simulink model "unifiedModelEdit"  (R2023b)
settings: Solver=FixedStepAuto  StartTime=0.0  StopTime=inf  RelTol=1e-3  EnableMultiTasking=on
libraries: vexarmcortexlib x25, vexcommonlib x6
settings Model: Creator=carol  LastModifiedBy=behja
settings SolverCC: AutoInsertRateTranBlk=on
settings DataIOCC: LimitDataPoints=on  SignalLoggingSaveFormat=ModelDataLogs  ReturnWorkspaceOutputs=off
settings OptimizationCC: ExpressionDepthLimit=2147483647  LifeSpan=Inf  MaxStackSize=64  EfficientTunableParamExpr=on
settings DebuggingCC: UnderspecifiedInitializationDetection=Classic  MergeDetectMultiDrivingBlocksExec=none  InheritedTsInSrcMsg=none  FcnCallInpInsideContextMsg=warning  StateNameClashWarn=warning  SFUnexpectedBacktrackingDiag=warning  SFNoUnconditionalDefaultTransitionDiag=warning  SFExecutionAtInitializationDiag=none  ArithmeticOperatorsInVariantConditions=warning
settings HardwareCC: ProdBitPerPointer=32  ProdBitPerSizeT=32  ProdBitPerPtrDiffT=32  ProdLargestAtomicInteger=Long  ProdLargestAtomicFloat=Double  ProdIntDivRoundTo=Undefined  ProdWordSize=32  ProdHWDeviceType=ARM Compatible->ARM Cortex
settings ModelReferenceCC: EnableRefExpFcnMdlSchedulingChecks=on  PropagateSignalLabelsOutOfModel=off
settings SFSimCC: MATLABDynamicMemAlloc=off  CustomCodeUndefinedFunction=UseInterfaceOnly
settings RTWCC: Description=Embedded Coder  SystemTargetFile=ert.tlc  HardwareBoard=ARM Cortex-based VEX Microcontroller  TemplateMakefile=ert_default_tmf  Toolchain=GNU Tools for VEX ARM Cortex
settings CodeAppCC: IgnoreCustomStorageClasses=off  CustomSymbolStrType=$N$R$M  StateflowObjectComments=on  InternalIdentifier=Classic
settings ERTTargetCC: CodeReplacementLibrary=GCC ARM Cortex-M3  MultiwordLength=2048  ConvertIfToSwitch=off  SuppressUnreachableDefaultCases=off

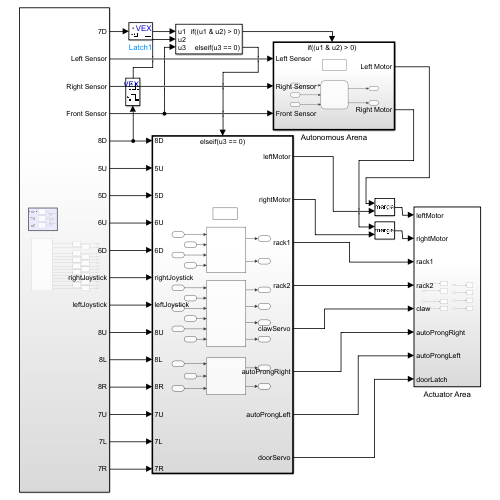
[thumbnail: Simulink's stored preview of the top-level diagram]
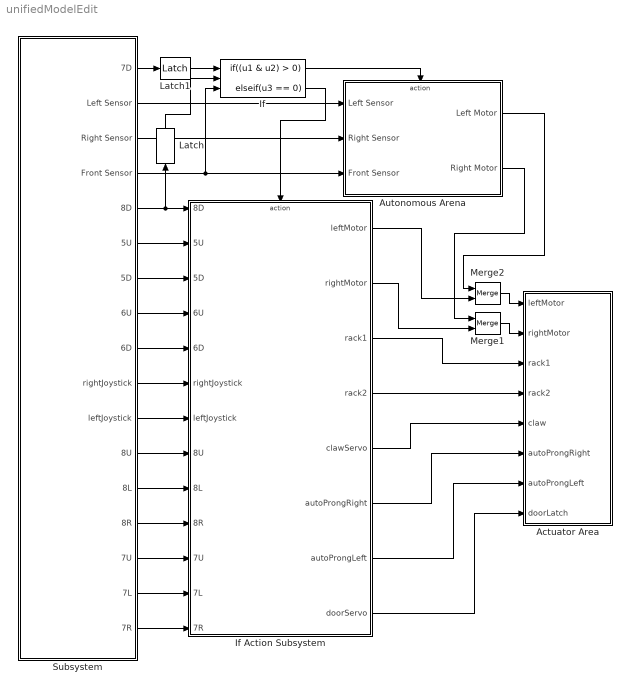
== system unifiedModelEdit ==
  Actuator Area : Subsystem
  Autonomous Arena : Subsystem  TreatAsAtomicUnit=on
  If : If  NumInputs=3  IfExpression=(u1 & u2) > 0  ElseIfExpressions=u3 == 0  ShowElse=off
  If Action Subsystem : Subsystem  TreatAsAtomicUnit=on
  Latch : vexcommonlib/Latch  output0=off  BlockPlatform=vexarmcortex
      settings: LibrarySourceBlock=vexarmcortexlib/Utilities/Latch
  Latch1 : vexcommonlib/Latch  output0=off  BlockPlatform=vexarmcortex
      settings: LibrarySourceBlock=vexarmcortexlib/Utilities/Latch
  Merge1 : Merge
  Merge2 : Merge
  Subsystem : Subsystem
  wires:
  Subsystem/3(Right Sensor) -> Autonomous Arena/2(Right Sensor)
  Subsystem/4(Front Sensor) -> If/3, Autonomous Arena/3(Front Sensor)
  If Action Subsystem/8(doorServo) -> Actuator Area/8(doorLatch)
  Subsystem/2(Left Sensor) -> Autonomous Arena/1(Left Sensor)
  Subsystem/5(8D) -> Latch/1, If Action Subsystem/1(8D)
  If Action Subsystem/5(clawServo) -> Actuator Area/5(claw)
  If Action Subsystem/3(rack1) -> Actuator Area/3(rack1)
  If Action Subsystem/6(autoProngRight) -> Actuator Area/6(autoProngRight)
  If Action Subsystem/4(rack2) -> Actuator Area/4(rack2)
  If Action Subsystem/7(autoProngLeft) -> Actuator Area/7(autoProngLeft)
  Subsystem/17(7R) -> If Action Subsystem/13(7R)
  Subsystem/16(7L) -> If Action Subsystem/12(7L)
  Subsystem/15(7U) -> If Action Subsystem/11(7U)
  Subsystem/14(8R) -> If Action Subsystem/10(8R)
  Subsystem/13(8L) -> If Action Subsystem/9(8L)
  Subsystem/12(8U) -> If Action Subsystem/8(8U)
  Subsystem/11(leftJoystick) -> If Action Subsystem/7(leftJoystick)
  Subsystem/10(rightJoystick) -> If Action Subsystem/6(rightJoystick)
  Subsystem/9(6D) -> If Action Subsystem/5(6D)
  Subsystem/8(6U) -> If Action Subsystem/4(6U)
  Subsystem/7(5D) -> If Action Subsystem/3(5D)
  Subsystem/6(5U) -> If Action Subsystem/2(5U)
  Merge1/1 -> Actuator Area/2(rightMotor)
  Merge2/1 -> Actuator Area/1(leftMotor)
  Autonomous Arena/1(Left Motor) -> Merge2/1
  If Action Subsystem/1(leftMotor) -> Merge2/2
  Autonomous Arena/2(Right Motor) -> Merge1/1
  If Action Subsystem/2(rightMotor) -> Merge1/2
  If/2 -> If Action Subsystem/Action
  If/1 -> Autonomous Arena/Action
  Latch/1 -> If/2
  Subsystem/1(7D) -> Latch1/1
  Latch1/1 -> If/1

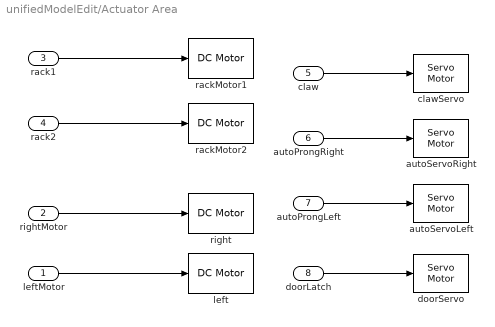
== system unifiedModelEdit/Actuator Area ==
  leftMotor : Inport
  rightMotor : Inport  Port=2
  rack1 : Inport  Port=3
  rack2 : Inport  Port=4
  claw : Inport  Port=5
  autoProngRight : Inport  Port=6
  autoProngLeft : Inport  Port=7
  doorLatch : Inport  Port=8
  autoServoLeft : vexarmcortexlib/Actuators/Servo Motor  motor=4  scaleFactor=60/127  SimulationOut=off
  autoServoRight : vexarmcortexlib/Actuators/Servo Motor  motor=7  scaleFactor=60/127  SimulationOut=off
  clawServo : vexarmcortexlib/Actuators/Servo Motor  motor=3  scaleFactor=60/127  SimulationOut=off
  doorServo : vexarmcortexlib/Actuators/Servo Motor  motor=8  scaleFactor=60/127  SimulationOut=off
  left : vexarmcortexlib/Actuators/DC Motor  motor=9  scaleFactor=1/13.5  SimulationOut=off
  rackMotor1 : vexarmcortexlib/Actuators/DC Motor  motor=5  scaleFactor=1/13.5  SimulationOut=off
  rackMotor2 : vexarmcortexlib/Actuators/DC Motor  motor=6  scaleFactor=1/13.5  SimulationOut=off
  right : vexarmcortexlib/Actuators/DC Motor  motor=2  scaleFactor=1/13.5  SimulationOut=off
  wires:
  leftMotor/1 -> left/1
  autoProngLeft/1 -> autoServoLeft/1
  rack1/1 -> rackMotor1/1
  rightMotor/1 -> right/1
  autoProngRight/1 -> autoServoRight/1
  doorLatch/1 -> doorServo/1
  claw/1 -> clawServo/1
  rack2/1 -> rackMotor2/1

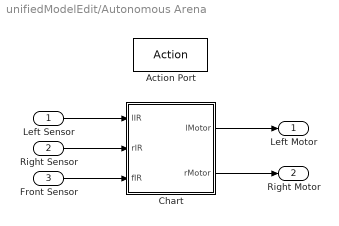
== system unifiedModelEdit/Autonomous Arena ==
  Left Sensor : Inport
  Right Sensor : Inport  Port=2
  Front Sensor : Inport  Port=3
  Action Port : ActionPort  ActionPortLabel=if((u1 & u2) > 0)
  Chart : Stateflow chart  TreatAsAtomicUnit=on
      settings: PortSchema="{\"entries\":[{\"content\":{\"sides\":[{\"content\":{\"connectorIds\":[\"In2\",\"In3\",\"In1\"]},\"type\":\"ConnectorPlacement.EquallySpacedRectSide\",\"uuid\":\"247074c7-d082-4199-9f42-5ee7f9b2f2c5\"},{\"content\":{\"connectorIds\":[\"Out1\",\"Out2\"],\"side\":\"RIGHT\"},\"type\":\"ConnectorPlacement.EquallySpacedRectSide\",\"uuid\":\"36e2493d-b1f5-4e64-901d-97da90bd168d\"},{\"content\":{\"side\":\"TOP\"},\"type\":\"ConnectorPlacement.EquallySpacedRectSide\",\"uuid\":\"46c427ed-bb7b-4aa4-a673-b474e6d6a53a\"}]},\"type\":\"ConnectorPlacement.EquallySpacedConnector\",\"uuid\":\"23614380-3184-4867-9eb4-661b2749fd08\"}],\"packageUris\":[\"http://schema.mathworks.com/mf0/Connector/R2020b\"],\"version\":\"1.0\"}"
  Left Motor : Outport
  Right Motor : Outport  Port=2
  wires:
  Left Sensor/1 -> Chart/2(lIR)
  Front Sensor/1 -> Chart/1(fIR)
  Right Sensor/1 -> Chart/3(rIR)
  Chart/1(lMotor) -> Left Motor/1
  Chart/2(rMotor) -> Right Motor/1

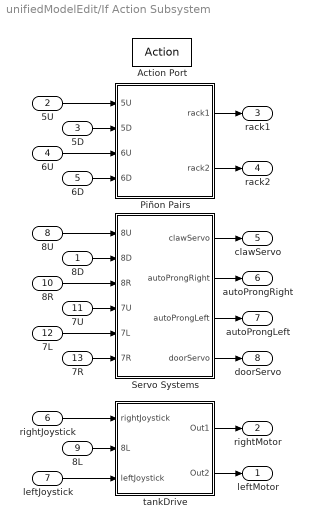
== system unifiedModelEdit/If Action Subsystem ==
  8D : Inport
  5U : Inport  Port=2
  5D : Inport  Port=3
  6U : Inport  Port=4
  6D : Inport  Port=5
  rightJoystick : Inport  Port=6
  leftJoystick : Inport  Port=7
  8U : Inport  Port=8
  8L : Inport  Port=9
  8R : Inport  Port=10
  7U : Inport  Port=11
  7L : Inport  Port=12
  7R : Inport  Port=13
  Action Port : ActionPort  ActionPortLabel=elseif(u3 == 0)
  Piñon Pairs : Subsystem
  Servo Systems : Subsystem
  tankDrive : Subsystem
  leftMotor : Outport
  rightMotor : Outport  Port=2
  rack1 : Outport  Port=3
  rack2 : Outport  Port=4
  clawServo : Outport  Port=5
  autoProngRight : Outport  Port=6
  autoProngLeft : Outport  Port=7
  doorServo : Outport  Port=8
  wires:
  Servo Systems/2(autoProngRight) -> autoProngRight/1
  Servo Systems/4(doorServo) -> doorServo/1
  Servo Systems/3(autoProngLeft) -> autoProngLeft/1
  Servo Systems/1(clawServo) -> clawServo/1
  7U/1 -> Servo Systems/4(7U)
  8D/1 -> Servo Systems/2(8D)
  Piñon Pairs/1(rack1) -> rack1/1
  8U/1 -> Servo Systems/1(8U)
  7R/1 -> Servo Systems/6(7R)
  6U/1 -> Piñon Pairs/3(6U)
  Piñon Pairs/2(rack2) -> rack2/1
  6D/1 -> Piñon Pairs/4(6D)
  7L/1 -> Servo Systems/5(7L)
  5U/1 -> Piñon Pairs/1(5U)
  8R/1 -> Servo Systems/3(8R)
  5D/1 -> Piñon Pairs/2(5D)
  rightJoystick/1 -> tankDrive/1(rightJoystick)
  8L/1 -> tankDrive/2("8L ")
  leftJoystick/1 -> tankDrive/3(leftJoystick)
  tankDrive/1(Out1) -> rightMotor/1
  tankDrive/2(Out2) -> leftMotor/1

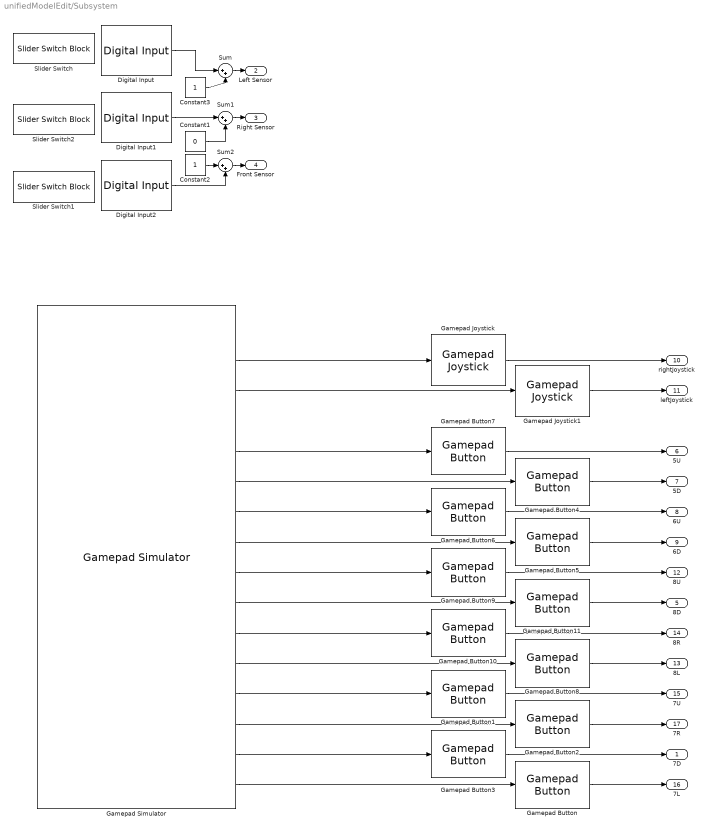
== system unifiedModelEdit/Subsystem ==
  Constant1 : Constant  Value=0
  Constant2 : Constant
  Constant3 : Constant
  Digital Input : vexarmcortexlib/Sensors/Digital Input  inChan=2  SimulationIn=off  SampleTime=0.2
  Digital Input1 : vexarmcortexlib/Sensors/Digital Input  inChan=11  SimulationIn=off  SampleTime=0.2
  Digital Input2 : vexarmcortexlib/Sensors/Digital Input  inChan=6  SimulationIn=off  SampleTime=0.2
  Gamepad Button : vexarmcortexlib/Gamepad/Gamepad Button  joystick=1  chan=7  button56=Up  button78=Left  SimulationIn=on  SampleTime=0.02
  Gamepad Button1 : vexarmcortexlib/Gamepad/Gamepad Button  joystick=1  chan=7  button56=Up  button78=Up  SimulationIn=on  SampleTime=0.02
  Gamepad Button10 : vexarmcortexlib/Gamepad/Gamepad Button  joystick=1  chan=8  button56=Up  button78=Right  SimulationIn=on  SampleTime=0.02
  Gamepad Button11 : vexarmcortexlib/Gamepad/Gamepad Button  joystick=1  chan=8  button56=Up  button78=Down  SimulationIn=on  SampleTime=0.02
  Gamepad Button2 : vexarmcortexlib/Gamepad/Gamepad Button  joystick=1  chan=7  button56=Up  button78=Right  SimulationIn=on  SampleTime=0.02
  Gamepad Button3 : vexarmcortexlib/Gamepad/Gamepad Button  joystick=1  chan=7  button56=Up  button78=Down  SimulationIn=on  SampleTime=0.02
  Gamepad Button4 : vexarmcortexlib/Gamepad/Gamepad Button  joystick=1  chan=5  button56=Down  button78=Down  SimulationIn=on  SampleTime=0.02
  Gamepad Button5 : vexarmcortexlib/Gamepad/Gamepad Button  joystick=1  chan=6  button56=Down  button78=Down  SimulationIn=on  SampleTime=0.02
  Gamepad Button6 : vexarmcortexlib/Gamepad/Gamepad Button  joystick=1  chan=6  button56=Up  button78=Down  SimulationIn=on  SampleTime=0.02
  Gamepad Button7 : vexarmcortexlib/Gamepad/Gamepad Button  joystick=1  chan=5  button56=Up  button78=Down  SimulationIn=on  SampleTime=0.02
  Gamepad Button8 : vexarmcortexlib/Gamepad/Gamepad Button  joystick=1  chan=8  button56=Up  button78=Left  SimulationIn=on  SampleTime=0.02
  Gamepad Button9 : vexarmcortexlib/Gamepad/Gamepad Button  joystick=1  chan=8  button56=Up  button78=Up  SimulationIn=on  SampleTime=0.02
  Gamepad Joystick : vexarmcortexlib/Gamepad/Gamepad Joystick  joystick=1  chan=2  SimulationIn=on  SampleTime=0.02
  Gamepad Joystick1 : vexarmcortexlib/Gamepad/Gamepad Joystick  joystick=1  chan=3  SimulationIn=on  SampleTime=0.02
  Gamepad Simulator : vexcommonlib/Gamepad Simulator  WhichPad=XBox Gamepad  JoyId=1  BlockPlatform=vexarmcortex
      settings: LibrarySourceBlock=vexarmcortexlib/Utilities/Gamepad Simulator
  Slider Switch : SliderSwitchBlock
      settings: Values={{'Off', 'On'}, [0 1]}
  Slider Switch1 : SliderSwitchBlock
      settings: Values={{'Off', 'On'}, [0 1]}
  Slider Switch2 : SliderSwitchBlock
      settings: Values={{'Off', 'On'}, [0 1]}
  Sum : Sum  Inputs=|++
  Sum1 : Sum  Inputs=|++
  Sum2 : Sum  Inputs=|++
  7D : Outport
  Left Sensor : Outport  Port=2
  Right Sensor : Outport  Port=3
  Front Sensor : Outport  Port=4
  8D : Outport  Port=5
  5U : Outport  Port=6
  5D : Outport  Port=7
  6U : Outport  Port=8
  6D : Outport  Port=9
  rightJoystick : Outport  Port=10
  leftJoystick : Outport  Port=11
  8U : Outport  Port=12
  8L : Outport  Port=13
  8R : Outport  Port=14
  7U : Outport  Port=15
  7L : Outport  Port=16
  7R : Outport  Port=17
  wires:
  Gamepad Simulator/15 -> Gamepad Button3/1
  Gamepad Simulator/9 -> Gamepad Button9/1
  Gamepad Simulator/12 -> Gamepad Button8/1
  Gamepad Button7/1 -> 5U/1
  Gamepad Button3/1 -> 7D/1
  Gamepad Simulator/14 -> Gamepad Button2/1
  Gamepad Button2/1 -> 7R/1
  Gamepad Simulator/7 -> Gamepad Button6/1
  Gamepad Simulator/16 -> Gamepad Button/1
  Gamepad Simulator/8 -> Gamepad Button5/1
  Gamepad Simulator/6 -> Gamepad Button4/1
  Gamepad Simulator/5 -> Gamepad Button7/1
  Gamepad Simulator/11 -> Gamepad Button10/1
  Gamepad Button10/1 -> 8R/1
  Gamepad Simulator/13 -> Gamepad Button1/1
  Gamepad Simulator/10 -> Gamepad Button11/1
  Gamepad Button8/1 -> 8L/1
  Gamepad Button9/1 -> 8U/1
  Gamepad Button5/1 -> 6D/1
  Gamepad Button/1 -> 7L/1
  Gamepad Button11/1 -> 8D/1
  Gamepad Button1/1 -> 7U/1
  Gamepad Button4/1 -> 5D/1
  Gamepad Button6/1 -> 6U/1
  Gamepad Simulator/2 -> Gamepad Joystick/1
  Gamepad Simulator/3 -> Gamepad Joystick1/1
  Digital Input2/1 -> Sum2/2
  Constant3/1 -> Sum/2
  Digital Input/1 -> Sum/1
  Constant1/1 -> Sum1/2
  Constant2/1 -> Sum2/1
  Digital Input1/1 -> Sum1/1
  Sum2/1 -> Front Sensor/1
  Sum1/1 -> Right Sensor/1
  Sum/1 -> Left Sensor/1
  Gamepad Joystick/1 -> rightJoystick/1
  Gamepad Joystick1/1 -> leftJoystick/1

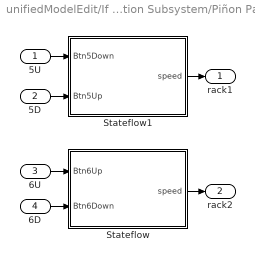
== system unifiedModelEdit/If Action Subsystem/Piñon Pairs ==
  5U : Inport
  5D : Inport  Port=2
  6U : Inport  Port=3
  6D : Inport  Port=4
  Stateflow : Stateflow chart  TreatAsAtomicUnit=on
  Stateflow1 : Stateflow chart  TreatAsAtomicUnit=on
  rack1 : Outport
  rack2 : Outport  Port=2
  wires:
  6U/1 -> Stateflow/1(Btn6Up)
  6D/1 -> Stateflow/2(Btn6Down)
  Stateflow/1(speed) -> rack2/1
  Stateflow1/1(speed) -> rack1/1
  5U/1 -> Stateflow1/1(Btn5Down)
  5D/1 -> Stateflow1/2(Btn5Up)

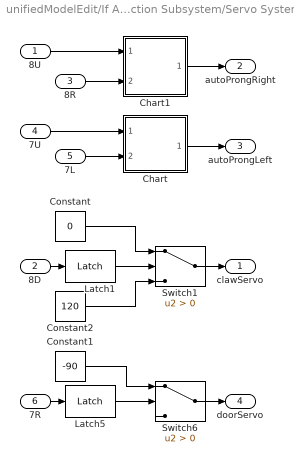
== system unifiedModelEdit/If Action Subsystem/Servo Systems ==
  8U : Inport
  8D : Inport  Port=2
  8R : Inport  Port=3
  7U : Inport  Port=4
  7L : Inport  Port=5
  7R : Inport  Port=6
  Chart : Stateflow chart  TreatAsAtomicUnit=on
  Chart1 : Stateflow chart  TreatAsAtomicUnit=on
  Constant : Constant  Value=0
  Constant1 : Constant  Value=-90
  Constant2 : Constant  Value=120
  Latch1 : vexcommonlib/Latch  output0=off  BlockPlatform=vexarmcortex
      settings: LibrarySourceBlock=vexarmcortexlib/Utilities/Latch
  Latch5 : vexcommonlib/Latch  output0=off  BlockPlatform=vexarmcortex
      settings: LibrarySourceBlock=vexarmcortexlib/Utilities/Latch
  Switch1 : Switch  Criteria=u2 > Threshold  SaturateOnIntegerOverflow=off  InputSameDT=off
  Switch6 : Switch  Criteria=u2 > Threshold  SaturateOnIntegerOverflow=off  InputSameDT=off
  clawServo : Outport
  autoProngRight : Outport  Port=2
  autoProngLeft : Outport  Port=3
  doorServo : Outport  Port=4
  wires:
  Constant1/1 -> Switch6/1
  Switch6/1 -> doorServo/1
  Switch1/1 -> clawServo/1
  8D/1 -> Latch1/1
  Constant2/1 -> Switch1/3
  Constant/1 -> Switch1/1
  Latch5/1 -> Switch6/2
  7R/1 -> Latch5/1
  Chart/1(angle) -> autoProngLeft/1
  7L/1 -> Chart/2(Btn7Left)
  7U/1 -> Chart/1(Btn7Up)
  Chart1/1(angle) -> autoProngRight/1
  8R/1 -> Chart1/2(Btn8Right)
  8U/1 -> Chart1/1(Btn8Up)
  Latch1/1 -> Switch1/2

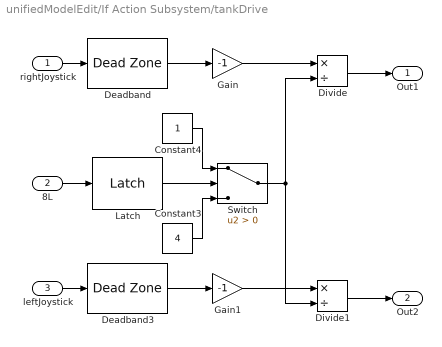
== system unifiedModelEdit/If Action Subsystem/tankDrive ==
  rightJoystick : Inport
  "8L " : Inport  Port=2
  leftJoystick : Inport  Port=3
  Constant3 : Constant  Value=4
  Constant4 : Constant
  Deadband : DeadZone  LowerValue=-9  UpperValue=9
  Deadband3 : DeadZone  LowerValue=-9  UpperValue=9
  Divide : Product  Inputs=*/
  Divide1 : Product  Inputs=*/
  Gain : Gain  Gain=-1
  Gain1 : Gain  Gain=-1
  Latch : vexcommonlib/Latch  output0=off  BlockPlatform=vexarmcortex
      settings: LibrarySourceBlock=vexarmcortexlib/Utilities/Latch
  Switch : Switch  Criteria=u2 > Threshold  SaturateOnIntegerOverflow=off  InputSameDT=off
  Out1 : Outport
  Out2 : Outport  Port=2
  wires:
  Constant4/1 -> Switch/1
  Constant3/1 -> Switch/3
  Divide1/1 -> Out2/1
  Latch/1 -> Switch/2
  Gain/1 -> Divide/1
  Gain1/1 -> Divide1/1
  Deadband3/1 -> Gain1/1
  Deadband/1 -> Gain/1
  Switch/1 -> Divide1/2, Divide/2
  rightJoystick/1 -> Deadband/1
  Divide/1 -> Out1/1
  "8L "/1 -> Latch/1
  leftJoystick/1 -> Deadband3/1

== stateflow chart unifiedModelEdit/If Action Subsystem/Servo Systems/Chart ==
  state neutral
    angle=0;
  state buffer
    angle=0;
  state negative90
    angle=-90;
  state positive90
    angle=90;
  (default) -> neutral
  neutral -> negative90 [order 1] : [Btn7Left==1 && Btn7Up==0]
  neutral -> positive90 [order 2] : [Btn7Up==1 && Btn7Left==0]
  buffer -> neutral : [after(7,sec)]
  negative90 -> buffer [order 1] : [Btn7Left==1 && Btn7Up==1]
  positive90 -> buffer [order 1] : [Btn7Up==1 && Btn7Left==1]
  negative90 -> positive90 [order 2] : [Btn7Left==0 && Btn7Up==1]
  positive90 -> negative90 [order 2] : [Btn7Up==0 && Btn7Left==1]
  data: Btn7Up input; Btn7Left input; angle output

== stateflow chart unifiedModelEdit/If Action Subsystem/Piñon Pairs/Stateflow ==
  state rackIN
    entry:
    speed=-127;
  state STOPPED
    entry:
    speed=0;
  state rackOUT
    entry:
    speed=127;
  (default) -> STOPPED
  STOPPED -> rackOUT [order 2] : [Btn6Down==0 && Btn6Up==1]
  STOPPED -> rackIN [order 1] : [Btn6Down==1 && Btn6Down==0]
  rackIN -> STOPPED [order 1] : [Btn6Down==0]
  rackOUT -> STOPPED [order 1] : [Btn6Up==0]
  rackIN -> STOPPED [order 2] : [Btn6Down==1 && Btn6Up==1]
  rackOUT -> STOPPED [order 2] : [Btn6Down==1 && Btn6Up==1]
  data: Btn6Up input; Btn6Down input; speed output

== stateflow chart unifiedModelEdit/If Action Subsystem/Piñon Pairs/Stateflow1 ==
  state rackIN
    entry:
    speed=-127;
  state STOPPED
    entry:
    speed=0;
  state rackOUT
    entry:
    speed=127;
  (default) -> STOPPED
  STOPPED -> rackOUT [order 2] : [Btn5Down==0 && Btn5Up==1]
  STOPPED -> rackIN [order 1] : [Btn5Down==1 && Btn5Down==0]
  rackIN -> STOPPED [order 1] : [Btn5Down==0]
  rackOUT -> STOPPED [order 1] : [Btn5Up==0]
  rackIN -> STOPPED [order 2] : [Btn5Down==1 && Btn5Up==1]
  rackOUT -> STOPPED [order 2] : [Btn5Down==1 && Btn5Up==1]
  data: speed output; Btn5Down input; Btn5Up input

== stateflow chart unifiedModelEdit/If Action Subsystem/Servo Systems/Chart1 ==
  state neutral
    angle=0;
  state buffer
    angle=0;
  state negative90
    angle=-90;
  state positive90
    angle=90;
  (default) -> neutral
  neutral -> negative90 [order 1] : [Btn8Right==1 && Btn8Up==0]
  neutral -> positive90 [order 2] : [Btn8Up==1 && Btn8Right==0]
  buffer -> neutral : [after(7,sec)]
  positive90 -> buffer [order 1] : [Btn8Up==1 && Btn8Right==1]
  negative90 -> buffer [order 1] : [Btn8Right==1 && Btn8Up==1]
  negative90 -> positive90 [order 2] : [Btn8Right==0 && Btn8Up==1]
  positive90 -> negative90 [order 2] : [Btn8Up==0 && Btn8Right==1]
  data: angle output; Btn8Up input; Btn8Right input

== stateflow chart unifiedModelEdit/Autonomous Arena/Chart ==
  state Follow
    Forward;
  state Middle
    lMotor = 0;
    rMotor = 0;
  state Start
    brainDetect = 0;
    slow = 1;
  Middle -> Follow : [brainDetect == 0]
  (default) -> Start
  Start -> Middle
  Follow -> Middle : [after(1,sec)&&brainDetect == 1]
  data: fIR input; lIR input; rIR input; lMotor output [-127..127] =50; rMotor output [-127..127] =50; brainDetect local [0..1] =0; slow local
  function Forward:
    | function Forward
    | 
    | init();
    | 
    | lIREQ0 = false;
    | rIREQ0 = false;
    | fIREQ0 = false;
    | 
    | 
    | % Left IR is equal to 0 should be 1
    | 
    | lIREQ0 = logical(lIR == 0);
    | 
    | % Right IR is equal to 0 should be 0
    | 
    | rIREQ0 = logical(rIR == 0);
    | 
    | % Front IR is equal to 0
    | 
    | fIREQ0 = logical(fIR == 0);
    | 
    | if (~lIREQ0 && rIREQ0 && ~fIREQ0)
    |     A5();
    | elseif (lIREQ0 && ~rIREQ0 && ~fIREQ0)
    |     A2();
    | elseif (lIREQ0 && rIREQ0 && ~fIREQ0)
    |     A2();
    | elseif (~lIREQ0 && ~rIREQ0 && ~fIREQ0)
    |     A3();
    | elseif (~lIREQ0 && ~rIREQ0 && fIREQ0)
    |     A4();
    | elseif (lIREQ0 && ~rIREQ0 && fIREQ0)
    |     A4();
    | elseif (lIREQ0 && rIREQ0 && fIREQ0)
    |     A4();
    | else % Default
    |     A4();
    | end
    | 
    | function init()
    | 
    | % Initial Speed
    | 
    | lMotor = 50/slow;
    | rMotor = 50/slow;
    | 
    | function A2()
    | 
    | % Left IR is seeing white - turn Left
    | 
    | lMotor = 25/slow;
    | 
    | function A3()
    | 
    | % Right IR is seeing black - turn Right
    | 
    | rMotor = 25/slow;
    | 
    | function A4()
    | 
    | % fIR is seeing the brain and the sensors are alighned - Stop
    | 
    | rMotor = 0;
    | lMotor = 0;
    | brainDetect = 1;
    | 
    | function A5()
    | 
    | % Everything is good
    | 
    | rMotor = 50/slow;
    | rMotor = 50/slow;
